simulink model "POModel"  (R2016a)
settings: Solver=VariableStepAuto  StartTime=0.0  StopTime=tEnd  RelTol=1e-3
values from neighbouring files (symbols this model uses):
  A = [-1 1 1;1 -2 0;0 1 -3]    [ExampleActuator.m]    (also in ExamplePIUIO.m = [-2 0 1;0 -1 1;1 2 -3]; NewExampleActuator.m; Simulation.m; SinousidPIUIO.m)
  Aa = [A,zeros(n,r);zeros(r,n),Md]    [Simulation.m]
  B = [1;1;0]    [ExampleActuator.m]    (also in ExamplePIUIO.m = [1;0;1]; NewExampleActuator.m; Simulation.m; SinousidPIUIO.m)
  Ba = [B;zeros(r,m)]    [Simulation.m]
  C = [1 0 0;0 1 0]    [ExampleActuator.m]    (also in ExamplePIUIO.m = [1 2 3;0 1 2]; NewExampleActuator.m = [1 0 1;0 1 0]; Simulation.m = [1 0 1;0 1 0]; SinousidPIUIO.m = [1 0 1;0 1 0])
  Ca = [C,zeros(p,r)]    [Simulation.m]
  d0 = [4;5]    [Simulation.m]
  Ed = [1;0;0]    [ExampleActuator.m]    (also in ExamplePIUIO.m = [1;1;0]; NewExampleActuator.m; Simulation.m; SinousidPIUIO.m = [1;0;1])
  La = Pa\Ya    [POfinder.m]
  Md = [-1 0;0 -1]    [Simulation.m]
  x0 = [1;2;3]    [ExampleActuator.m]    (also in ExamplePIUIO.m; NewExampleActuator.m; Simulation.m; SinousidPIUIO.m)
  xhat0 = [2;1;1]    [ExamplePIUIO.m]    (also in Simulation.m = [.1;.2;.3;.4;.5]; SinousidPIUIO.m)
settings Model: Creator=amirreza513  LastModifiedBy=amirreza513

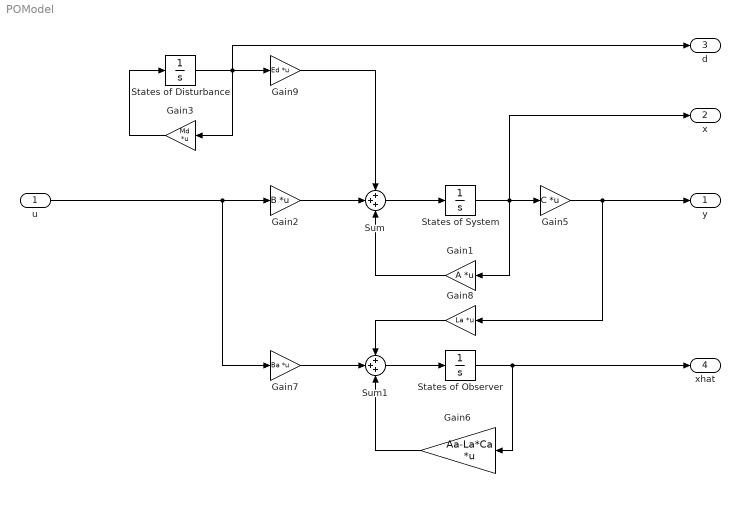
== system POModel ==
  u : Inport
  Gain1 : Gain  Gain=A  Multiplication=Matrix(K*u) (u vector)
  Gain2 : Gain  Gain=B  Multiplication=Matrix(K*u) (u vector)
  Gain3 : Gain  Gain=Md  Multiplication=Matrix(K*u) (u vector)
  Gain5 : Gain  Gain=C  Multiplication=Matrix(K*u) (u vector)
  Gain6 : Gain  Gain=Aa-La*Ca  Multiplication=Matrix(K*u) (u vector)
  Gain7 : Gain  Gain=Ba  Multiplication=Matrix(K*u) (u vector)
  Gain8 : Gain  Gain=La  Multiplication=Matrix(K*u) (u vector)
  Gain9 : Gain  Gain=Ed  Multiplication=Matrix(K*u) (u vector)
  States of Disturbance : Integrator  InitialCondition=d0
  States of Observer : Integrator  InitialCondition=xhat0
  States of System : Integrator  InitialCondition=x0
  Sum : Sum  Inputs=+++
  Sum1 : Sum  Inputs=+++
  y : Outport
  x : Outport  Port=2
  d : Outport  Port=3
  xhat : Outport  Port=4
  wires:
  States of System/1 -> x/1, Gain5/1, Gain1/1
  u/1 -> Gain7/1, Gain2/1
  Sum/1 -> States of System/1
  Gain5/1 -> Gain8/1, y/1
  Gain3/1 -> States of Disturbance/1
  States of Disturbance/1 -> d/1, Gain3/1, Gain9/1
  Gain2/1 -> Sum/2
  Gain1/1 -> Sum/3
  Gain8/1 -> Sum1/1
  Sum1/1 -> States of Observer/1
  Gain7/1 -> Sum1/2
  States of Observer/1 -> xhat/1, Gain6/1
  Gain6/1 -> Sum1/3
  Gain9/1 -> Sum/1
